simulink model "ch7example5"  (Simulink 5.0)
settings: Solver=FixedStepDiscrete  StartTime=0.0  StopTime=20.0  FixedStep=1/10  RelTol=1e-3
libraries: commrandsrc2 x1, dspswit3 x1, simulink x1
settings Model: LastModifiedBy=shaoyubin

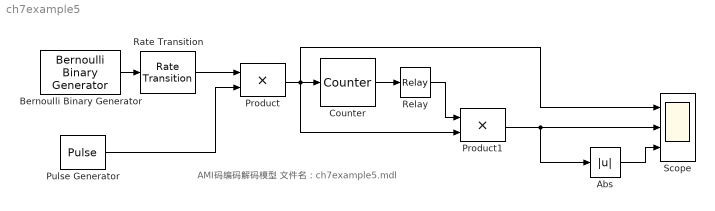
== system ch7example5 ==
  note: AMI码编码解码模型
      | 文件名：ch7example5.mdl
  Abs : Abs  SaturateOnIntegerOverflow=on
  Bernoulli Binary Generator : commrandsrc2/Bernoulli Binary Generator  P=0.5  seed=61  Ts=1  frameBased=off  sampPerFrame=1  orient=off
  Counter : dspswit3/Counter  Direction=Up  CountEvent=Rising edge  CounterSize=User defined  MaxCount=1  InitialCount=0  Output=Count  HitValue=32  ResetInput=off  SamplesPerFrame=1  Ts=1  CntDtype=Double  HitDtype=Logical
  Product : Product  SaturateOnIntegerOverflow=on
  Product1 : Product  SaturateOnIntegerOverflow=on
  Pulse Generator : DiscretePulseGenerator  Period=10  PulseWidth=5  SampleTime=1/10
  Rate Transition : simulink/Signal Attributes/Rate Transition  DataIntegrity=on  DeterministicTransfer=on  TransitionType=Slow to fast  InitCond=0
  Relay : Relay  OnSwitchValue=0.5  OffSwitchValue=0.5  OffOutputValue=-1
  Scope : Scope  NumInputPorts=3
      settings: TickLabels=off  YMin=-2~-2~-2  YMax=2~2~2
  wires:
  Bernoulli Binary Generator/1 -> Rate Transition/1
  Pulse Generator/1 -> Product/2
  Rate Transition/1 -> Product/1
  Product/1 -> Counter/1, Product1/2, Scope/1
  Counter/1 -> Relay/1
  Relay/1 -> Product1/1
  Product1/1 -> Scope/2, Abs/1
  Abs/1 -> Scope/3
